simulink model "doubleIntegratorControlUncons"  (R2015b)
settings: Solver=ode8  StartTime=0.0  StopTime=2  FixedStep=0.01  RelTol=1e-3
settings Model: Creator=E183308  LastModifiedBy=E183308

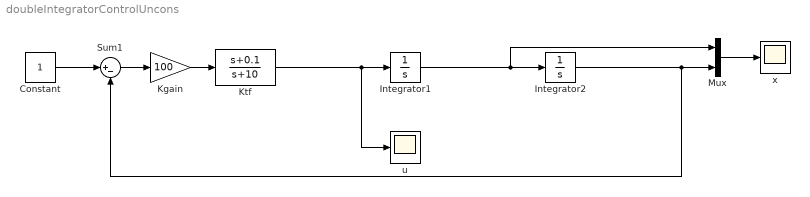
== system doubleIntegratorControlUncons ==
  Constant : Constant
  Integrator1 : Integrator  UpperSaturationLimit=3  LowerSaturationLimit=-3
  Integrator2 : Integrator
  Kgain : Gain  Gain=100
  Ktf : TransferFcn  Numerator=[1 0.1]  Denominator=[1 10]
  Mux : Mux  Inputs=2
  Sum1 : Sum  Inputs=|+-
  u : Scope
  x : Scope
  wires:
  Constant/1 -> Sum1/1
  Kgain/1 -> Ktf/1
  Sum1/1 -> Kgain/1
  Mux/1 -> x/1
  Integrator1/1 -> Mux/1, Integrator2/1
  Integrator2/1 -> Mux/2, Sum1/2
  Ktf/1 -> u/1, Integrator1/1
